simulink model "IOControls"  (R2019b)
settings: configuration reference "ConfigSet_IOControls_Reference" (kept outside this file)
model workspace (MAT data in the model file):
  SampleTime = 0.05
libraries: IOStateMachinesLib x274, SignalGeneratorsLib x1, simulink x1
(part 6 of 10)

== system IOControls/ForEachVehicle/IOControls/Non-CabControl/CircuitBreakersofEDB/ILCB2 ==
  note: States:
      | Tripped
      | Set
  MCBControl : Inport  OutDataTypeStr=Bus: BD_IOControls_In_MCBControl
  Initialise : Inport  Port=2
  Bus Selector : BusSelector  OutputSignals=Value,Mode,InitVal,InternalRequest,Inhibit,TripRequest
  ILCB2-MCB : IOStateMachinesLib/MCB  InitSource=internal  InitState=InitState  OffStateValue=OffStateValue  OnStateValue=OnStateValue
      settings: SourceProductName=IO State Machines
  InputState : Outport  VectorParamsAs1DForOutWhenUnconnected=off
  MCBTripState : Outport  Port=2  VectorParamsAs1DForOutWhenUnconnected=off
  wires:
  ILCB2-MCB/2 -> MCBTripState/1
  Bus Selector/6 -> ILCB2-MCB/7  "<TripRequest>"
  MCBControl/1 -> Bus Selector/1
  Bus Selector/1 -> ILCB2-MCB/1  "<Value>"
  Bus Selector/2 -> ILCB2-MCB/2  "<Mode>"
  Bus Selector/3 -> ILCB2-MCB/3  "<InitVal>"
  Bus Selector/4 -> ILCB2-MCB/5  "<InternalRequest>"
  Bus Selector/5 -> ILCB2-MCB/6  "<Inhibit>"
  ILCB2-MCB/1 -> InputState/1
  Initialise/1 -> ILCB2-MCB/4

== system IOControls/ForEachVehicle/IOControls/Non-CabControl/CircuitBreakersofEDB/LDICB ==
  note: States:
      | Tripped
      | Set
  MCBControl : Inport  OutDataTypeStr=Bus: BD_IOControls_In_MCBControl
  Initialise : Inport  Port=2
  Bus Selector : BusSelector  OutputSignals=Value,Mode,InitVal,InternalRequest,Inhibit,TripRequest
  LDICB-MCB : IOStateMachinesLib/MCB  InitSource=internal  InitState=InitState  OffStateValue=OffStateValue  OnStateValue=OnStateValue
      settings: SourceProductName=IO State Machines
  InputState : Outport  VectorParamsAs1DForOutWhenUnconnected=off
  MCBTripState : Outport  Port=2  VectorParamsAs1DForOutWhenUnconnected=off
  wires:
  LDICB-MCB/2 -> MCBTripState/1
  Bus Selector/6 -> LDICB-MCB/7  "<TripRequest>"
  MCBControl/1 -> Bus Selector/1
  Bus Selector/1 -> LDICB-MCB/1  "<Value>"
  Bus Selector/2 -> LDICB-MCB/2  "<Mode>"
  Bus Selector/3 -> LDICB-MCB/3  "<InitVal>"
  Bus Selector/4 -> LDICB-MCB/5  "<InternalRequest>"
  Bus Selector/5 -> LDICB-MCB/6  "<Inhibit>"
  LDICB-MCB/1 -> InputState/1
  Initialise/1 -> LDICB-MCB/4

== system IOControls/ForEachVehicle/IOControls/Non-CabControl/CircuitBreakersofEDB/LDLCB ==
  note: States:
      | Tripped
      | Set
  MCBControl : Inport  OutDataTypeStr=Bus: BD_IOControls_In_MCBControl
  Initialise : Inport  Port=2
  Bus Selector : BusSelector  OutputSignals=Value,Mode,InitVal,InternalRequest,Inhibit,TripRequest
  LDLCB-MCB : IOStateMachinesLib/MCB  InitSource=internal  InitState=InitState  OffStateValue=OffStateValue  OnStateValue=OnStateValue
      settings: SourceProductName=IO State Machines
  InputState : Outport  VectorParamsAs1DForOutWhenUnconnected=off
  MCBTripState : Outport  Port=2  VectorParamsAs1DForOutWhenUnconnected=off
  wires:
  LDLCB-MCB/2 -> MCBTripState/1
  Bus Selector/6 -> LDLCB-MCB/7  "<TripRequest>"
  MCBControl/1 -> Bus Selector/1
  Bus Selector/1 -> LDLCB-MCB/1  "<Value>"
  Bus Selector/2 -> LDLCB-MCB/2  "<Mode>"
  Bus Selector/3 -> LDLCB-MCB/3  "<InitVal>"
  Bus Selector/4 -> LDLCB-MCB/5  "<InternalRequest>"
  Bus Selector/5 -> LDLCB-MCB/6  "<Inhibit>"
  LDLCB-MCB/1 -> InputState/1
  Initialise/1 -> LDLCB-MCB/4

== system IOControls/ForEachVehicle/IOControls/Non-CabControl/CircuitBreakersofEDB/LDRCB ==
  note: States:
      | Tripped
      | Set
  MCBControl : Inport  OutDataTypeStr=Bus: BD_IOControls_In_MCBControl
  Initialise : Inport  Port=2
  Bus Selector : BusSelector  OutputSignals=Value,Mode,InitVal,InternalRequest,Inhibit,TripRequest
  LDRCB-MCB : IOStateMachinesLib/MCB  InitSource=internal  InitState=InitState  OffStateValue=OffStateValue  OnStateValue=OnStateValue
      settings: SourceProductName=IO State Machines
  InputState : Outport  VectorParamsAs1DForOutWhenUnconnected=off
  MCBTripState : Outport  Port=2  VectorParamsAs1DForOutWhenUnconnected=off
  wires:
  LDRCB-MCB/2 -> MCBTripState/1
  Bus Selector/6 -> LDRCB-MCB/7  "<TripRequest>"
  MCBControl/1 -> Bus Selector/1
  Bus Selector/1 -> LDRCB-MCB/1  "<Value>"
  Bus Selector/2 -> LDRCB-MCB/2  "<Mode>"
  Bus Selector/3 -> LDRCB-MCB/3  "<InitVal>"
  Bus Selector/4 -> LDRCB-MCB/5  "<InternalRequest>"
  Bus Selector/5 -> LDRCB-MCB/6  "<Inhibit>"
  LDRCB-MCB/1 -> InputState/1
  Initialise/1 -> LDRCB-MCB/4

== system IOControls/ForEachVehicle/IOControls/Non-CabControl/CircuitBreakersofEDB/MLCB ==
  note: States:
      | Tripped
      | Set
  MCBControl : Inport  OutDataTypeStr=Bus: BD_IOControls_In_MCBControl
  Initialise : Inport  Port=2
  Bus Selector : BusSelector  OutputSignals=Value,Mode,InitVal,InternalRequest,Inhibit,TripRequest
  MLCB-MCB : IOStateMachinesLib/MCB  InitSource=internal  InitState=InitState  OffStateValue=OffStateValue  OnStateValue=OnStateValue
      settings: SourceProductName=IO State Machines
  InputState : Outport  VectorParamsAs1DForOutWhenUnconnected=off
  MCBTripState : Outport  Port=2  VectorParamsAs1DForOutWhenUnconnected=off
  wires:
  MLCB-MCB/2 -> MCBTripState/1
  Bus Selector/6 -> MLCB-MCB/7  "<TripRequest>"
  MCBControl/1 -> Bus Selector/1
  Bus Selector/1 -> MLCB-MCB/1  "<Value>"
  Bus Selector/2 -> MLCB-MCB/2  "<Mode>"
  Bus Selector/3 -> MLCB-MCB/3  "<InitVal>"
  Bus Selector/4 -> MLCB-MCB/5  "<InternalRequest>"
  Bus Selector/5 -> MLCB-MCB/6  "<Inhibit>"
  MLCB-MCB/1 -> InputState/1
  Initialise/1 -> MLCB-MCB/4

== system IOControls/ForEachVehicle/IOControls/Non-CabControl/CircuitBreakersofEDB/MMCB ==
  note: States:
      | Tripped
      | Set
  MCBControl : Inport  OutDataTypeStr=Bus: BD_IOControls_In_MCBControl
  Initialise : Inport  Port=2
  Bus Selector : BusSelector  OutputSignals=Value,Mode,InitVal,InternalRequest,Inhibit,TripRequest
  MMCB-MCB : IOStateMachinesLib/MCB  InitSource=internal  InitState=InitState  OffStateValue=OffStateValue  OnStateValue=OnStateValue
      settings: SourceProductName=IO State Machines
  InputState : Outport  VectorParamsAs1DForOutWhenUnconnected=off
  MCBTripState : Outport  Port=2  VectorParamsAs1DForOutWhenUnconnected=off
  wires:
  MMCB-MCB/2 -> MCBTripState/1
  Bus Selector/6 -> MMCB-MCB/7  "<TripRequest>"
  MCBControl/1 -> Bus Selector/1
  Bus Selector/1 -> MMCB-MCB/1  "<Value>"
  Bus Selector/2 -> MMCB-MCB/2  "<Mode>"
  Bus Selector/3 -> MMCB-MCB/3  "<InitVal>"
  Bus Selector/4 -> MMCB-MCB/5  "<InternalRequest>"
  Bus Selector/5 -> MMCB-MCB/6  "<Inhibit>"
  MMCB-MCB/1 -> InputState/1
  Initialise/1 -> MMCB-MCB/4

== system IOControls/ForEachVehicle/IOControls/Non-CabControl/CircuitBreakersofEDB/MSOCB1 ==
  note: States:
      | Tripped
      | Set
  MCBControl : Inport  OutDataTypeStr=Bus: BD_IOControls_In_MCBControl
  Initialise : Inport  Port=2
  Bus Selector : BusSelector  OutputSignals=Value,Mode,InitVal,InternalRequest,Inhibit,TripRequest
  MSOCB1-MCB : IOStateMachinesLib/MCB  InitSource=internal  InitState=InitState  OffStateValue=OffStateValue  OnStateValue=OnStateValue
      settings: SourceProductName=IO State Machines
  InputState : Outport  VectorParamsAs1DForOutWhenUnconnected=off
  MCBTripState : Outport  Port=2  VectorParamsAs1DForOutWhenUnconnected=off
  wires:
  MSOCB1-MCB/2 -> MCBTripState/1
  Bus Selector/6 -> MSOCB1-MCB/7  "<TripRequest>"
  MCBControl/1 -> Bus Selector/1
  Bus Selector/1 -> MSOCB1-MCB/1  "<Value>"
  Bus Selector/2 -> MSOCB1-MCB/2  "<Mode>"
  Bus Selector/3 -> MSOCB1-MCB/3  "<InitVal>"
  Bus Selector/4 -> MSOCB1-MCB/5  "<InternalRequest>"
  Bus Selector/5 -> MSOCB1-MCB/6  "<Inhibit>"
  MSOCB1-MCB/1 -> InputState/1
  Initialise/1 -> MSOCB1-MCB/4

== system IOControls/ForEachVehicle/IOControls/Non-CabControl/CircuitBreakersofEDB/MSOCB2 ==
  note: States:
      | Tripped
      | Set
  MCBControl : Inport  OutDataTypeStr=Bus: BD_IOControls_In_MCBControl
  Initialise : Inport  Port=2
  Bus Selector : BusSelector  OutputSignals=Value,Mode,InitVal,InternalRequest,Inhibit,TripRequest
  MSOCB2-MCB : IOStateMachinesLib/MCB  InitSource=internal  InitState=InitState  OffStateValue=OffStateValue  OnStateValue=OnStateValue
      settings: SourceProductName=IO State Machines
  InputState : Outport  VectorParamsAs1DForOutWhenUnconnected=off
  MCBTripState : Outport  Port=2  VectorParamsAs1DForOutWhenUnconnected=off
  wires:
  MSOCB2-MCB/2 -> MCBTripState/1
  Bus Selector/6 -> MSOCB2-MCB/7  "<TripRequest>"
  MCBControl/1 -> Bus Selector/1
  Bus Selector/1 -> MSOCB2-MCB/1  "<Value>"
  Bus Selector/2 -> MSOCB2-MCB/2  "<Mode>"
  Bus Selector/3 -> MSOCB2-MCB/3  "<InitVal>"
  Bus Selector/4 -> MSOCB2-MCB/5  "<InternalRequest>"
  Bus Selector/5 -> MSOCB2-MCB/6  "<Inhibit>"
  MSOCB2-MCB/1 -> InputState/1
  Initialise/1 -> MSOCB2-MCB/4

== system IOControls/ForEachVehicle/IOControls/Non-CabControl/CircuitBreakersofEDB/MSOCB3 ==
  note: States:
      | Tripped
      | Set
  MCBControl : Inport  OutDataTypeStr=Bus: BD_IOControls_In_MCBControl
  Initialise : Inport  Port=2
  Bus Selector : BusSelector  OutputSignals=Value,Mode,InitVal,InternalRequest,Inhibit,TripRequest
  MSOCB3-MCB : IOStateMachinesLib/MCB  InitSource=internal  InitState=InitState  OffStateValue=OffStateValue  OnStateValue=OnStateValue
      settings: SourceProductName=IO State Machines
  InputState : Outport  VectorParamsAs1DForOutWhenUnconnected=off
  MCBTripState : Outport  Port=2  VectorParamsAs1DForOutWhenUnconnected=off
  wires:
  MSOCB3-MCB/2 -> MCBTripState/1
  Bus Selector/6 -> MSOCB3-MCB/7  "<TripRequest>"
  MCBControl/1 -> Bus Selector/1
  Bus Selector/1 -> MSOCB3-MCB/1  "<Value>"
  Bus Selector/2 -> MSOCB3-MCB/2  "<Mode>"
  Bus Selector/3 -> MSOCB3-MCB/3  "<InitVal>"
  Bus Selector/4 -> MSOCB3-MCB/5  "<InternalRequest>"
  Bus Selector/5 -> MSOCB3-MCB/6  "<Inhibit>"
  MSOCB3-MCB/1 -> InputState/1
  Initialise/1 -> MSOCB3-MCB/4

== system IOControls/ForEachVehicle/IOControls/Non-CabControl/CircuitBreakersofEDB/MSOCB4 ==
  note: States:
      | Tripped
      | Set
  MCBControl : Inport  OutDataTypeStr=Bus: BD_IOControls_In_MCBControl
  Initialise : Inport  Port=2
  Bus Selector : BusSelector  OutputSignals=Value,Mode,InitVal,InternalRequest,Inhibit,TripRequest
  MSOCB4-MCB : IOStateMachinesLib/MCB  InitSource=internal  InitState=InitState  OffStateValue=OffStateValue  OnStateValue=OnStateValue
      settings: SourceProductName=IO State Machines
  InputState : Outport  VectorParamsAs1DForOutWhenUnconnected=off
  MCBTripState : Outport  Port=2  VectorParamsAs1DForOutWhenUnconnected=off
  wires:
  MSOCB4-MCB/2 -> MCBTripState/1
  Bus Selector/6 -> MSOCB4-MCB/7  "<TripRequest>"
  MCBControl/1 -> Bus Selector/1
  Bus Selector/1 -> MSOCB4-MCB/1  "<Value>"
  Bus Selector/2 -> MSOCB4-MCB/2  "<Mode>"
  Bus Selector/3 -> MSOCB4-MCB/3  "<InitVal>"
  Bus Selector/4 -> MSOCB4-MCB/5  "<InternalRequest>"
  Bus Selector/5 -> MSOCB4-MCB/6  "<Inhibit>"
  MSOCB4-MCB/1 -> InputState/1
  Initialise/1 -> MSOCB4-MCB/4

== system IOControls/ForEachVehicle/IOControls/Non-CabControl/CircuitBreakersofEDB/MSOCB5 ==
  note: States:
      | Tripped
      | Set
  MCBControl : Inport  OutDataTypeStr=Bus: BD_IOControls_In_MCBControl
  Initialise : Inport  Port=2
  Bus Selector : BusSelector  OutputSignals=Value,Mode,InitVal,InternalRequest,Inhibit,TripRequest
  MSOCB5-MCB : IOStateMachinesLib/MCB  InitSource=internal  InitState=InitState  OffStateValue=OffStateValue  OnStateValue=OnStateValue
      settings: SourceProductName=IO State Machines
  InputState : Outport  VectorParamsAs1DForOutWhenUnconnected=off
  MCBTripState : Outport  Port=2  VectorParamsAs1DForOutWhenUnconnected=off
  wires:
  MSOCB5-MCB/2 -> MCBTripState/1
  Bus Selector/6 -> MSOCB5-MCB/7  "<TripRequest>"
  MCBControl/1 -> Bus Selector/1
  Bus Selector/1 -> MSOCB5-MCB/1  "<Value>"
  Bus Selector/2 -> MSOCB5-MCB/2  "<Mode>"
  Bus Selector/3 -> MSOCB5-MCB/3  "<InitVal>"
  Bus Selector/4 -> MSOCB5-MCB/5  "<InternalRequest>"
  Bus Selector/5 -> MSOCB5-MCB/6  "<Inhibit>"
  MSOCB5-MCB/1 -> InputState/1
  Initialise/1 -> MSOCB5-MCB/4

== system IOControls/ForEachVehicle/IOControls/Non-CabControl/CircuitBreakersofEDB/MTBM1CB ==
  note: States:
      | Tripped
      | Set
  MCBControl : Inport  OutDataTypeStr=Bus: BD_IOControls_In_MCBControl
  Initialise : Inport  Port=2
  Bus Selector : BusSelector  OutputSignals=Value,Mode,InitVal,InternalRequest,Inhibit,TripRequest
  MTBM1CB-MCB : IOStateMachinesLib/MCB  InitSource=internal  InitState=InitState  OffStateValue=OffStateValue  OnStateValue=OnStateValue
      settings: SourceProductName=IO State Machines
  InputState : Outport  VectorParamsAs1DForOutWhenUnconnected=off
  MCBTripState : Outport  Port=2  VectorParamsAs1DForOutWhenUnconnected=off
  wires:
  MTBM1CB-MCB/2 -> MCBTripState/1
  Bus Selector/6 -> MTBM1CB-MCB/7  "<TripRequest>"
  MCBControl/1 -> Bus Selector/1
  Bus Selector/1 -> MTBM1CB-MCB/1  "<Value>"
  Bus Selector/2 -> MTBM1CB-MCB/2  "<Mode>"
  Bus Selector/3 -> MTBM1CB-MCB/3  "<InitVal>"
  Bus Selector/4 -> MTBM1CB-MCB/5  "<InternalRequest>"
  Bus Selector/5 -> MTBM1CB-MCB/6  "<Inhibit>"
  MTBM1CB-MCB/1 -> InputState/1
  Initialise/1 -> MTBM1CB-MCB/4

== system IOControls/ForEachVehicle/IOControls/Non-CabControl/CircuitBreakersofEDB/MTBM2CB ==
  note: States:
      | Tripped
      | Set
  MCBControl : Inport  OutDataTypeStr=Bus: BD_IOControls_In_MCBControl
  Initialise : Inport  Port=2
  Bus Selector : BusSelector  OutputSignals=Value,Mode,InitVal,InternalRequest,Inhibit,TripRequest
  MTBM2CB-MCB : IOStateMachinesLib/MCB  InitSource=internal  InitState=InitState  OffStateValue=OffStateValue  OnStateValue=OnStateValue
      settings: SourceProductName=IO State Machines
  InputState : Outport  VectorParamsAs1DForOutWhenUnconnected=off
  MCBTripState : Outport  Port=2  VectorParamsAs1DForOutWhenUnconnected=off
  wires:
  MTBM2CB-MCB/2 -> MCBTripState/1
  Bus Selector/6 -> MTBM2CB-MCB/7  "<TripRequest>"
  MCBControl/1 -> Bus Selector/1
  Bus Selector/1 -> MTBM2CB-MCB/1  "<Value>"
  Bus Selector/2 -> MTBM2CB-MCB/2  "<Mode>"
  Bus Selector/3 -> MTBM2CB-MCB/3  "<InitVal>"
  Bus Selector/4 -> MTBM2CB-MCB/5  "<InternalRequest>"
  Bus Selector/5 -> MTBM2CB-MCB/6  "<Inhibit>"
  MTBM2CB-MCB/1 -> InputState/1
  Initialise/1 -> MTBM2CB-MCB/4

== system IOControls/ForEachVehicle/IOControls/Non-CabControl/CircuitBreakersofEDB/MTBMCCB ==
  note: States:
      | Tripped
      | Set
  MCBControl : Inport  OutDataTypeStr=Bus: BD_IOControls_In_MCBControl
  Initialise : Inport  Port=2
  Bus Selector : BusSelector  OutputSignals=Value,Mode,InitVal,InternalRequest,Inhibit,TripRequest
  MTBMCCB-MCB : IOStateMachinesLib/MCB  InitSource=internal  InitState=InitState  OffStateValue=OffStateValue  OnStateValue=OnStateValue
      settings: SourceProductName=IO State Machines
  InputState : Outport  VectorParamsAs1DForOutWhenUnconnected=off
  MCBTripState : Outport  Port=2  VectorParamsAs1DForOutWhenUnconnected=off
  wires:
  MTBMCCB-MCB/2 -> MCBTripState/1
  Bus Selector/6 -> MTBMCCB-MCB/7  "<TripRequest>"
  MCBControl/1 -> Bus Selector/1
  Bus Selector/1 -> MTBMCCB-MCB/1  "<Value>"
  Bus Selector/2 -> MTBMCCB-MCB/2  "<Mode>"
  Bus Selector/3 -> MTBMCCB-MCB/3  "<InitVal>"
  Bus Selector/4 -> MTBMCCB-MCB/5  "<InternalRequest>"
  Bus Selector/5 -> MTBMCCB-MCB/6  "<Inhibit>"
  MTBMCCB-MCB/1 -> InputState/1
  Initialise/1 -> MTBMCCB-MCB/4

== system IOControls/ForEachVehicle/IOControls/Non-CabControl/CircuitBreakersofEDB/MTOPCB ==
  note: States:
      | Tripped
      | Set
  MCBControl : Inport  OutDataTypeStr=Bus: BD_IOControls_In_MCBControl
  Initialise : Inport  Port=2
  Bus Selector : BusSelector  OutputSignals=Value,Mode,InitVal,InternalRequest,Inhibit,TripRequest
  MTOPCB-MCB : IOStateMachinesLib/MCB  InitSource=internal  InitState=InitState  OffStateValue=OffStateValue  OnStateValue=OnStateValue
      settings: SourceProductName=IO State Machines
  InputState : Outport  VectorParamsAs1DForOutWhenUnconnected=off
  MCBTripState : Outport  Port=2  VectorParamsAs1DForOutWhenUnconnected=off
  wires:
  MTOPCB-MCB/2 -> MCBTripState/1
  Bus Selector/6 -> MTOPCB-MCB/7  "<TripRequest>"
  MCBControl/1 -> Bus Selector/1
  Bus Selector/1 -> MTOPCB-MCB/1  "<Value>"
  Bus Selector/2 -> MTOPCB-MCB/2  "<Mode>"
  Bus Selector/3 -> MTOPCB-MCB/3  "<InitVal>"
  Bus Selector/4 -> MTOPCB-MCB/5  "<InternalRequest>"
  Bus Selector/5 -> MTOPCB-MCB/6  "<Inhibit>"
  MTOPCB-MCB/1 -> InputState/1
  Initialise/1 -> MTOPCB-MCB/4

== system IOControls/ForEachVehicle/IOControls/Non-CabControl/CircuitBreakersofEDB/NBCB ==
  note: States:
      | Tripped
      | Set
  MCBControl : Inport  OutDataTypeStr=Bus: BD_IOControls_In_MCBControl
  Initialise : Inport  Port=2
  Bus Selector : BusSelector  OutputSignals=Value,Mode,InitVal,InternalRequest,Inhibit,TripRequest
  NBCB-MCB : IOStateMachinesLib/MCB  InitSource=internal  InitState=InitState  OffStateValue=OffStateValue  OnStateValue=OnStateValue
      settings: SourceProductName=IO State Machines
  InputState : Outport  VectorParamsAs1DForOutWhenUnconnected=off
  MCBTripState : Outport  Port=2  VectorParamsAs1DForOutWhenUnconnected=off
  wires:
  NBCB-MCB/2 -> MCBTripState/1
  Bus Selector/6 -> NBCB-MCB/7  "<TripRequest>"
  MCBControl/1 -> Bus Selector/1
  Bus Selector/1 -> NBCB-MCB/1  "<Value>"
  Bus Selector/2 -> NBCB-MCB/2  "<Mode>"
  Bus Selector/3 -> NBCB-MCB/3  "<InitVal>"
  Bus Selector/4 -> NBCB-MCB/5  "<InternalRequest>"
  Bus Selector/5 -> NBCB-MCB/6  "<Inhibit>"
  NBCB-MCB/1 -> InputState/1
  Initialise/1 -> NBCB-MCB/4

== system IOControls/ForEachVehicle/IOControls/Non-CabControl/CircuitBreakersofEDB/NVICB ==
  note: States:
      | Tripped
      | Set
  MCBControl : Inport  OutDataTypeStr=Bus: BD_IOControls_In_MCBControl
  Initialise : Inport  Port=2
  Bus Selector : BusSelector  OutputSignals=Value,Mode,InitVal,InternalRequest,Inhibit,TripRequest
  NVICB-MCB : IOStateMachinesLib/MCB  InitSource=internal  InitState=InitState  OffStateValue=OffStateValue  OnStateValue=OnStateValue
      settings: SourceProductName=IO State Machines
  InputState : Outport  VectorParamsAs1DForOutWhenUnconnected=off
  MCBTripState : Outport  Port=2  VectorParamsAs1DForOutWhenUnconnected=off
  wires:
  NVICB-MCB/2 -> MCBTripState/1
  Bus Selector/6 -> NVICB-MCB/7  "<TripRequest>"
  MCBControl/1 -> Bus Selector/1
  Bus Selector/1 -> NVICB-MCB/1  "<Value>"
  Bus Selector/2 -> NVICB-MCB/2  "<Mode>"
  Bus Selector/3 -> NVICB-MCB/3  "<InitVal>"
  Bus Selector/4 -> NVICB-MCB/5  "<InternalRequest>"
  Bus Selector/5 -> NVICB-MCB/6  "<Inhibit>"
  NVICB-MCB/1 -> InputState/1
  Initialise/1 -> NVICB-MCB/4

== system IOControls/ForEachVehicle/IOControls/Non-CabControl/CircuitBreakersofEDB/OCCB1 ==
  note: States:
      | Tripped
      | Set
  MCBControl : Inport  OutDataTypeStr=Bus: BD_IOControls_In_MCBControl
  Initialise : Inport  Port=2
  Bus Selector : BusSelector  OutputSignals=Value,Mode,InitVal,InternalRequest,Inhibit,TripRequest
  OCCB1-MCB : IOStateMachinesLib/MCB  InitSource=internal  InitState=InitState  OffStateValue=OffStateValue  OnStateValue=OnStateValue
      settings: SourceProductName=IO State Machines
  InputState : Outport  VectorParamsAs1DForOutWhenUnconnected=off
  MCBTripState : Outport  Port=2  VectorParamsAs1DForOutWhenUnconnected=off
  wires:
  OCCB1-MCB/2 -> MCBTripState/1
  Bus Selector/6 -> OCCB1-MCB/7  "<TripRequest>"
  MCBControl/1 -> Bus Selector/1
  Bus Selector/1 -> OCCB1-MCB/1  "<Value>"
  Bus Selector/2 -> OCCB1-MCB/2  "<Mode>"
  Bus Selector/3 -> OCCB1-MCB/3  "<InitVal>"
  Bus Selector/4 -> OCCB1-MCB/5  "<InternalRequest>"
  Bus Selector/5 -> OCCB1-MCB/6  "<Inhibit>"
  OCCB1-MCB/1 -> InputState/1
  Initialise/1 -> OCCB1-MCB/4

== system IOControls/ForEachVehicle/IOControls/Non-CabControl/CircuitBreakersofEDB/OCCB2 ==
  note: States:
      | Tripped
      | Set
  MCBControl : Inport  OutDataTypeStr=Bus: BD_IOControls_In_MCBControl
  Initialise : Inport  Port=2
  Bus Selector : BusSelector  OutputSignals=Value,Mode,InitVal,InternalRequest,Inhibit,TripRequest
  OCCB2-MCB : IOStateMachinesLib/MCB  InitSource=internal  InitState=InitState  OffStateValue=OffStateValue  OnStateValue=OnStateValue
      settings: SourceProductName=IO State Machines
  InputState : Outport  VectorParamsAs1DForOutWhenUnconnected=off
  MCBTripState : Outport  Port=2  VectorParamsAs1DForOutWhenUnconnected=off
  wires:
  OCCB2-MCB/2 -> MCBTripState/1
  Bus Selector/6 -> OCCB2-MCB/7  "<TripRequest>"
  MCBControl/1 -> Bus Selector/1
  Bus Selector/1 -> OCCB2-MCB/1  "<Value>"
  Bus Selector/2 -> OCCB2-MCB/2  "<Mode>"
  Bus Selector/3 -> OCCB2-MCB/3  "<InitVal>"
  Bus Selector/4 -> OCCB2-MCB/5  "<InternalRequest>"
  Bus Selector/5 -> OCCB2-MCB/6  "<Inhibit>"
  OCCB2-MCB/1 -> InputState/1
  Initialise/1 -> OCCB2-MCB/4

== system IOControls/ForEachVehicle/IOControls/Non-CabControl/CircuitBreakersofEDB/ODDCB ==
  note: States:
      | Tripped
      | Set
  MCBControl : Inport  OutDataTypeStr=Bus: BD_IOControls_In_MCBControl
  Initialise : Inport  Port=2
  Bus Selector : BusSelector  OutputSignals=Value,Mode,InitVal,InternalRequest,Inhibit,TripRequest
  ODDCB-MCB : IOStateMachinesLib/MCB  InitSource=internal  InitState=InitState  OffStateValue=OffStateValue  OnStateValue=OnStateValue
      settings: SourceProductName=IO State Machines
  InputState : Outport  VectorParamsAs1DForOutWhenUnconnected=off
  MCBTripState : Outport  Port=2  VectorParamsAs1DForOutWhenUnconnected=off
  wires:
  ODDCB-MCB/2 -> MCBTripState/1
  Bus Selector/6 -> ODDCB-MCB/7  "<TripRequest>"
  MCBControl/1 -> Bus Selector/1
  Bus Selector/1 -> ODDCB-MCB/1  "<Value>"
  Bus Selector/2 -> ODDCB-MCB/2  "<Mode>"
  Bus Selector/3 -> ODDCB-MCB/3  "<InitVal>"
  Bus Selector/4 -> ODDCB-MCB/5  "<InternalRequest>"
  Bus Selector/5 -> ODDCB-MCB/6  "<Inhibit>"
  ODDCB-MCB/1 -> InputState/1
  Initialise/1 -> ODDCB-MCB/4

== system IOControls/ForEachVehicle/IOControls/Non-CabControl/CircuitBreakersofEDB/ORDCOS ==
  note: States:
      | Normal
      | Cutout
  InputControl : Inport  OutDataTypeStr=Bus: BD_IOControls_In_InputControl
  Initialise : Inport  Port=2
  Bus Selector : BusSelector  OutputSignals=Value,Mode,InitVal,InternalRequest,Inhibit
  ORDCOS-Toggle : IOStateMachinesLib/Toggle  InitSource=internal  InitState=InitState  OffStateValue=OffStateValue  OnStateValue=OnStateValue
      settings: SourceProductName=IO State Machines
  InputState : Outport  VectorParamsAs1DForOutWhenUnconnected=off
  wires:
  Initialise/1 -> ORDCOS-Toggle/4
  ORDCOS-Toggle/1 -> InputState/1
  Bus Selector/5 -> ORDCOS-Toggle/6  "<Inhibit>"
  Bus Selector/4 -> ORDCOS-Toggle/5  "<InternalRequest>"
  Bus Selector/3 -> ORDCOS-Toggle/3  "<InitVal>"
  Bus Selector/2 -> ORDCOS-Toggle/2  "<Mode>"
  Bus Selector/1 -> ORDCOS-Toggle/1  "<Value>"
  InputControl/1 -> Bus Selector/1

== system IOControls/ForEachVehicle/IOControls/Non-CabControl/CircuitBreakersofEDB/PADCB ==
  note: States:
      | Tripped
      | Set
  MCBControl : Inport  OutDataTypeStr=Bus: BD_IOControls_In_MCBControl
  Initialise : Inport  Port=2
  Bus Selector : BusSelector  OutputSignals=Value,Mode,InitVal,InternalRequest,Inhibit,TripRequest
  PADCB-MCB : IOStateMachinesLib/MCB  InitSource=internal  InitState=InitState  OffStateValue=OffStateValue  OnStateValue=OnStateValue
      settings: SourceProductName=IO State Machines
  InputState : Outport  VectorParamsAs1DForOutWhenUnconnected=off
  MCBTripState : Outport  Port=2  VectorParamsAs1DForOutWhenUnconnected=off
  wires:
  PADCB-MCB/2 -> MCBTripState/1
  Bus Selector/6 -> PADCB-MCB/7  "<TripRequest>"
  MCBControl/1 -> Bus Selector/1
  Bus Selector/1 -> PADCB-MCB/1  "<Value>"
  Bus Selector/2 -> PADCB-MCB/2  "<Mode>"
  Bus Selector/3 -> PADCB-MCB/3  "<InitVal>"
  Bus Selector/4 -> PADCB-MCB/5  "<InternalRequest>"
  Bus Selector/5 -> PADCB-MCB/6  "<Inhibit>"
  PADCB-MCB/1 -> InputState/1
  Initialise/1 -> PADCB-MCB/4

== system IOControls/ForEachVehicle/IOControls/Non-CabControl/CircuitBreakersofEDB/PANCB ==
  note: States:
      | Tripped
      | Set
  MCBControl : Inport  OutDataTypeStr=Bus: BD_IOControls_In_MCBControl
  Initialise : Inport  Port=2
  Bus Selector : BusSelector  OutputSignals=Value,Mode,InitVal,InternalRequest,Inhibit,TripRequest
  PANCB-MCB : IOStateMachinesLib/MCB  InitSource=internal  InitState=InitState  OffStateValue=OffStateValue  OnStateValue=OnStateValue
      settings: SourceProductName=IO State Machines
  InputState : Outport  VectorParamsAs1DForOutWhenUnconnected=off
  MCBTripState : Outport  Port=2  VectorParamsAs1DForOutWhenUnconnected=off
  wires:
  PANCB-MCB/2 -> MCBTripState/1
  Bus Selector/6 -> PANCB-MCB/7  "<TripRequest>"
  MCBControl/1 -> Bus Selector/1
  Bus Selector/1 -> PANCB-MCB/1  "<Value>"
  Bus Selector/2 -> PANCB-MCB/2  "<Mode>"
  Bus Selector/3 -> PANCB-MCB/3  "<InitVal>"
  Bus Selector/4 -> PANCB-MCB/5  "<InternalRequest>"
  Bus Selector/5 -> PANCB-MCB/6  "<Inhibit>"
  PANCB-MCB/1 -> InputState/1
  Initialise/1 -> PANCB-MCB/4

== system IOControls/ForEachVehicle/IOControls/Non-CabControl/CircuitBreakersofEDB/PBCB ==
  note: States:
      | Tripped
      | Set
  MCBControl : Inport  OutDataTypeStr=Bus: BD_IOControls_In_MCBControl
  Initialise : Inport  Port=2
  Bus Selector : BusSelector  OutputSignals=Value,Mode,InitVal,InternalRequest,Inhibit,TripRequest
  PBCB-MCB : IOStateMachinesLib/MCB  InitSource=internal  InitState=InitState  OffStateValue=OffStateValue  OnStateValue=OnStateValue
      settings: SourceProductName=IO State Machines
  InputState : Outport  VectorParamsAs1DForOutWhenUnconnected=off
  MCBTripState : Outport  Port=2  VectorParamsAs1DForOutWhenUnconnected=off
  wires:
  PBCB-MCB/2 -> MCBTripState/1
  Bus Selector/6 -> PBCB-MCB/7  "<TripRequest>"
  MCBControl/1 -> Bus Selector/1
  Bus Selector/1 -> PBCB-MCB/1  "<Value>"
  Bus Selector/2 -> PBCB-MCB/2  "<Mode>"
  Bus Selector/3 -> PBCB-MCB/3  "<InitVal>"
  Bus Selector/4 -> PBCB-MCB/5  "<InternalRequest>"
  Bus Selector/5 -> PBCB-MCB/6  "<Inhibit>"
  PBCB-MCB/1 -> InputState/1
  Initialise/1 -> PBCB-MCB/4

== system IOControls/ForEachVehicle/IOControls/Non-CabControl/CircuitBreakersofEDB/PISCB1 ==
  note: States:
      | Tripped
      | Set
  MCBControl : Inport  OutDataTypeStr=Bus: BD_IOControls_In_MCBControl
  Initialise : Inport  Port=2
  Bus Selector : BusSelector  OutputSignals=Value,Mode,InitVal,InternalRequest,Inhibit,TripRequest
  PISCB1-MCB : IOStateMachinesLib/MCB  InitSource=internal  InitState=InitState  OffStateValue=OffStateValue  OnStateValue=OnStateValue
      settings: SourceProductName=IO State Machines
  InputState : Outport  VectorParamsAs1DForOutWhenUnconnected=off
  MCBTripState : Outport  Port=2  VectorParamsAs1DForOutWhenUnconnected=off
  wires:
  PISCB1-MCB/2 -> MCBTripState/1
  Bus Selector/6 -> PISCB1-MCB/7  "<TripRequest>"
  MCBControl/1 -> Bus Selector/1
  Bus Selector/1 -> PISCB1-MCB/1  "<Value>"
  Bus Selector/2 -> PISCB1-MCB/2  "<Mode>"
  Bus Selector/3 -> PISCB1-MCB/3  "<InitVal>"
  Bus Selector/4 -> PISCB1-MCB/5  "<InternalRequest>"
  Bus Selector/5 -> PISCB1-MCB/6  "<Inhibit>"
  PISCB1-MCB/1 -> InputState/1
  Initialise/1 -> PISCB1-MCB/4

== system IOControls/ForEachVehicle/IOControls/Non-CabControl/CircuitBreakersofEDB/PISCB2 ==
  note: States:
      | Tripped
      | Set
  MCBControl : Inport  OutDataTypeStr=Bus: BD_IOControls_In_MCBControl
  Initialise : Inport  Port=2
  Bus Selector : BusSelector  OutputSignals=Value,Mode,InitVal,InternalRequest,Inhibit,TripRequest
  PISCB2-MCB : IOStateMachinesLib/MCB  InitSource=internal  InitState=InitState  OffStateValue=OffStateValue  OnStateValue=OnStateValue
      settings: SourceProductName=IO State Machines
  InputState : Outport  VectorParamsAs1DForOutWhenUnconnected=off
  MCBTripState : Outport  Port=2  VectorParamsAs1DForOutWhenUnconnected=off
  wires:
  PISCB2-MCB/2 -> MCBTripState/1
  Bus Selector/6 -> PISCB2-MCB/7  "<TripRequest>"
  MCBControl/1 -> Bus Selector/1
  Bus Selector/1 -> PISCB2-MCB/1  "<Value>"
  Bus Selector/2 -> PISCB2-MCB/2  "<Mode>"
  Bus Selector/3 -> PISCB2-MCB/3  "<InitVal>"
  Bus Selector/4 -> PISCB2-MCB/5  "<InternalRequest>"
  Bus Selector/5 -> PISCB2-MCB/6  "<Inhibit>"
  PISCB2-MCB/1 -> InputState/1
  Initialise/1 -> PISCB2-MCB/4

== system IOControls/ForEachVehicle/IOControls/Non-CabControl/CircuitBreakersofEDB/POCB ==
  note: States:
      | Tripped
      | Set
  MCBControl : Inport  OutDataTypeStr=Bus: BD_IOControls_In_MCBControl
  Initialise : Inport  Port=2
  Bus Selector : BusSelector  OutputSignals=Value,Mode,InitVal,InternalRequest,Inhibit,TripRequest
  POCB-MCB : IOStateMachinesLib/MCB  InitSource=internal  InitState=InitState  OffStateValue=OffStateValue  OnStateValue=OnStateValue
      settings: SourceProductName=IO State Machines
  InputState : Outport  VectorParamsAs1DForOutWhenUnconnected=off
  MCBTripState : Outport  Port=2  VectorParamsAs1DForOutWhenUnconnected=off
  wires:
  POCB-MCB/2 -> MCBTripState/1
  Bus Selector/6 -> POCB-MCB/7  "<TripRequest>"
  MCBControl/1 -> Bus Selector/1
  Bus Selector/1 -> POCB-MCB/1  "<Value>"
  Bus Selector/2 -> POCB-MCB/2  "<Mode>"
  Bus Selector/3 -> POCB-MCB/3  "<InitVal>"
  Bus Selector/4 -> POCB-MCB/5  "<InternalRequest>"
  Bus Selector/5 -> POCB-MCB/6  "<Inhibit>"
  POCB-MCB/1 -> InputState/1
  Initialise/1 -> POCB-MCB/4

== system IOControls/ForEachVehicle/IOControls/Non-CabControl/CircuitBreakersofEDB/PPU1CB ==
  note: States:
      | Tripped
      | Set
  MCBControl : Inport  OutDataTypeStr=Bus: BD_IOControls_In_MCBControl
  Initialise : Inport  Port=2
  Bus Selector : BusSelector  OutputSignals=Value,Mode,InitVal,InternalRequest,Inhibit,TripRequest
  PPU1CB-MCB : IOStateMachinesLib/MCB  InitSource=internal  InitState=InitState  OffStateValue=OffStateValue  OnStateValue=OnStateValue
      settings: SourceProductName=IO State Machines
  InputState : Outport  VectorParamsAs1DForOutWhenUnconnected=off
  MCBTripState : Outport  Port=2  VectorParamsAs1DForOutWhenUnconnected=off
  wires:
  PPU1CB-MCB/2 -> MCBTripState/1
  Bus Selector/6 -> PPU1CB-MCB/7  "<TripRequest>"
  MCBControl/1 -> Bus Selector/1
  Bus Selector/1 -> PPU1CB-MCB/1  "<Value>"
  Bus Selector/2 -> PPU1CB-MCB/2  "<Mode>"
  Bus Selector/3 -> PPU1CB-MCB/3  "<InitVal>"
  Bus Selector/4 -> PPU1CB-MCB/5  "<InternalRequest>"
  Bus Selector/5 -> PPU1CB-MCB/6  "<Inhibit>"
  PPU1CB-MCB/1 -> InputState/1
  Initialise/1 -> PPU1CB-MCB/4

== system IOControls/ForEachVehicle/IOControls/Non-CabControl/CircuitBreakersofEDB/PPU2CB ==
  note: States:
      | Tripped
      | Set
  MCBControl : Inport  OutDataTypeStr=Bus: BD_IOControls_In_MCBControl
  Initialise : Inport  Port=2
  Bus Selector : BusSelector  OutputSignals=Value,Mode,InitVal,InternalRequest,Inhibit,TripRequest
  PPU2CB-MCB : IOStateMachinesLib/MCB  InitSource=internal  InitState=InitState  OffStateValue=OffStateValue  OnStateValue=OnStateValue
      settings: SourceProductName=IO State Machines
  InputState : Outport  VectorParamsAs1DForOutWhenUnconnected=off
  MCBTripState : Outport  Port=2  VectorParamsAs1DForOutWhenUnconnected=off
  wires:
  PPU2CB-MCB/2 -> MCBTripState/1
  Bus Selector/6 -> PPU2CB-MCB/7  "<TripRequest>"
  MCBControl/1 -> Bus Selector/1
  Bus Selector/1 -> PPU2CB-MCB/1  "<Value>"
  Bus Selector/2 -> PPU2CB-MCB/2  "<Mode>"
  Bus Selector/3 -> PPU2CB-MCB/3  "<InitVal>"
  Bus Selector/4 -> PPU2CB-MCB/5  "<InternalRequest>"
  Bus Selector/5 -> PPU2CB-MCB/6  "<Inhibit>"
  PPU2CB-MCB/1 -> InputState/1
  Initialise/1 -> PPU2CB-MCB/4

== system IOControls/ForEachVehicle/IOControls/Non-CabControl/CircuitBreakersofEDB/PPU3CB ==
  note: States:
      | Tripped
      | Set
  MCBControl : Inport  OutDataTypeStr=Bus: BD_IOControls_In_MCBControl
  Initialise : Inport  Port=2
  Bus Selector : BusSelector  OutputSignals=Value,Mode,InitVal,InternalRequest,Inhibit,TripRequest
  PPU3CB-MCB : IOStateMachinesLib/MCB  InitSource=internal  InitState=InitState  OffStateValue=OffStateValue  OnStateValue=OnStateValue
      settings: SourceProductName=IO State Machines
  InputState : Outport  VectorParamsAs1DForOutWhenUnconnected=off
  MCBTripState : Outport  Port=2  VectorParamsAs1DForOutWhenUnconnected=off
  wires:
  PPU3CB-MCB/2 -> MCBTripState/1
  Bus Selector/6 -> PPU3CB-MCB/7  "<TripRequest>"
  MCBControl/1 -> Bus Selector/1
  Bus Selector/1 -> PPU3CB-MCB/1  "<Value>"
  Bus Selector/2 -> PPU3CB-MCB/2  "<Mode>"
  Bus Selector/3 -> PPU3CB-MCB/3  "<InitVal>"
  Bus Selector/4 -> PPU3CB-MCB/5  "<InternalRequest>"
  Bus Selector/5 -> PPU3CB-MCB/6  "<Inhibit>"
  PPU3CB-MCB/1 -> InputState/1
  Initialise/1 -> PPU3CB-MCB/4

== system IOControls/ForEachVehicle/IOControls/Non-CabControl/CircuitBreakersofEDB/PTCB ==
  note: States:
      | Tripped
      | Set
  MCBControl : Inport  OutDataTypeStr=Bus: BD_IOControls_In_MCBControl
  Initialise : Inport  Port=2
  Bus Selector : BusSelector  OutputSignals=Value,Mode,InitVal,InternalRequest,Inhibit,TripRequest
  PTCB-MCB : IOStateMachinesLib/MCB  InitSource=internal  InitState=InitState  OffStateValue=OffStateValue  OnStateValue=OnStateValue
      settings: SourceProductName=IO State Machines
  InputState : Outport  VectorParamsAs1DForOutWhenUnconnected=off
  MCBTripState : Outport  Port=2  VectorParamsAs1DForOutWhenUnconnected=off
  wires:
  PTCB-MCB/2 -> MCBTripState/1
  Bus Selector/6 -> PTCB-MCB/7  "<TripRequest>"
  MCBControl/1 -> Bus Selector/1
  Bus Selector/1 -> PTCB-MCB/1  "<Value>"
  Bus Selector/2 -> PTCB-MCB/2  "<Mode>"
  Bus Selector/3 -> PTCB-MCB/3  "<InitVal>"
  Bus Selector/4 -> PTCB-MCB/5  "<InternalRequest>"
  Bus Selector/5 -> PTCB-MCB/6  "<Inhibit>"
  PTCB-MCB/1 -> InputState/1
  Initialise/1 -> PTCB-MCB/4

== system IOControls/ForEachVehicle/IOControls/Non-CabControl/CircuitBreakersofEDB/RIO1CB ==
  note: States:
      | Tripped
      | Set
  MCBControl : Inport  OutDataTypeStr=Bus: BD_IOControls_In_MCBControl
  Initialise : Inport  Port=2
  Bus Selector : BusSelector  OutputSignals=Value,Mode,InitVal,InternalRequest,Inhibit,TripRequest
  RIO1CB-MCB : IOStateMachinesLib/MCB  InitSource=internal  InitState=InitState  OffStateValue=OffStateValue  OnStateValue=OnStateValue
      settings: SourceProductName=IO State Machines
  InputState : Outport  VectorParamsAs1DForOutWhenUnconnected=off
  MCBTripState : Outport  Port=2  VectorParamsAs1DForOutWhenUnconnected=off
  wires:
  RIO1CB-MCB/2 -> MCBTripState/1
  Bus Selector/6 -> RIO1CB-MCB/7  "<TripRequest>"
  MCBControl/1 -> Bus Selector/1
  Bus Selector/1 -> RIO1CB-MCB/1  "<Value>"
  Bus Selector/2 -> RIO1CB-MCB/2  "<Mode>"
  Bus Selector/3 -> RIO1CB-MCB/3  "<InitVal>"
  Bus Selector/4 -> RIO1CB-MCB/5  "<InternalRequest>"
  Bus Selector/5 -> RIO1CB-MCB/6  "<Inhibit>"
  RIO1CB-MCB/1 -> InputState/1
  Initialise/1 -> RIO1CB-MCB/4

== system IOControls/ForEachVehicle/IOControls/Non-CabControl/CircuitBreakersofEDB/RIO2CB ==
  note: States:
      | Tripped
      | Set
  MCBControl : Inport  OutDataTypeStr=Bus: BD_IOControls_In_MCBControl
  Initialise : Inport  Port=2
  Bus Selector : BusSelector  OutputSignals=Value,Mode,InitVal,InternalRequest,Inhibit,TripRequest
  RIO2CB-MCB : IOStateMachinesLib/MCB  InitSource=internal  InitState=InitState  OffStateValue=OffStateValue  OnStateValue=OnStateValue
      settings: SourceProductName=IO State Machines
  InputState : Outport  VectorParamsAs1DForOutWhenUnconnected=off
  MCBTripState : Outport  Port=2  VectorParamsAs1DForOutWhenUnconnected=off
  wires:
  RIO2CB-MCB/2 -> MCBTripState/1
  Bus Selector/6 -> RIO2CB-MCB/7  "<TripRequest>"
  MCBControl/1 -> Bus Selector/1
  Bus Selector/1 -> RIO2CB-MCB/1  "<Value>"
  Bus Selector/2 -> RIO2CB-MCB/2  "<Mode>"
  Bus Selector/3 -> RIO2CB-MCB/3  "<InitVal>"
  Bus Selector/4 -> RIO2CB-MCB/5  "<InternalRequest>"
  Bus Selector/5 -> RIO2CB-MCB/6  "<Inhibit>"
  RIO2CB-MCB/1 -> InputState/1
  Initialise/1 -> RIO2CB-MCB/4

== system IOControls/ForEachVehicle/IOControls/Non-CabControl/CircuitBreakersofEDB/RPTCB ==
  note: States:
      | Tripped
      | Set
  MCBControl : Inport  OutDataTypeStr=Bus: BD_IOControls_In_MCBControl
  Initialise : Inport  Port=2
  Bus Selector : BusSelector  OutputSignals=Value,Mode,InitVal,InternalRequest,Inhibit,TripRequest
  RPTCB-MCB : IOStateMachinesLib/MCB  InitSource=internal  InitState=InitState  OffStateValue=OffStateValue  OnStateValue=OnStateValue
      settings: SourceProductName=IO State Machines
  InputState : Outport  VectorParamsAs1DForOutWhenUnconnected=off
  MCBTripState : Outport  Port=2  VectorParamsAs1DForOutWhenUnconnected=off
  wires:
  RPTCB-MCB/2 -> MCBTripState/1
  Bus Selector/6 -> RPTCB-MCB/7  "<TripRequest>"
  MCBControl/1 -> Bus Selector/1
  Bus Selector/1 -> RPTCB-MCB/1  "<Value>"
  Bus Selector/2 -> RPTCB-MCB/2  "<Mode>"
  Bus Selector/3 -> RPTCB-MCB/3  "<InitVal>"
  Bus Selector/4 -> RPTCB-MCB/5  "<InternalRequest>"
  Bus Selector/5 -> RPTCB-MCB/6  "<Inhibit>"
  RPTCB-MCB/1 -> InputState/1
  Initialise/1 -> RPTCB-MCB/4

== system IOControls/ForEachVehicle/IOControls/Non-CabControl/CircuitBreakersofEDB/RSACB ==
  note: States:
      | Tripped
      | Set
  MCBControl : Inport  OutDataTypeStr=Bus: BD_IOControls_In_MCBControl
  Initialise : Inport  Port=2
  Bus Selector : BusSelector  OutputSignals=Value,Mode,InitVal,InternalRequest,Inhibit,TripRequest
  RSACB-MCB : IOStateMachinesLib/MCB  InitSource=internal  InitState=InitState  OffStateValue=OffStateValue  OnStateValue=OnStateValue
      settings: SourceProductName=IO State Machines
  InputState : Outport  VectorParamsAs1DForOutWhenUnconnected=off
  MCBTripState : Outport  Port=2  VectorParamsAs1DForOutWhenUnconnected=off
  wires:
  RSACB-MCB/2 -> MCBTripState/1
  Bus Selector/6 -> RSACB-MCB/7  "<TripRequest>"
  MCBControl/1 -> Bus Selector/1
  Bus Selector/1 -> RSACB-MCB/1  "<Value>"
  Bus Selector/2 -> RSACB-MCB/2  "<Mode>"
  Bus Selector/3 -> RSACB-MCB/3  "<InitVal>"
  Bus Selector/4 -> RSACB-MCB/5  "<InternalRequest>"
  Bus Selector/5 -> RSACB-MCB/6  "<Inhibit>"
  RSACB-MCB/1 -> InputState/1
  Initialise/1 -> RSACB-MCB/4

== system IOControls/ForEachVehicle/IOControls/Non-CabControl/CircuitBreakersofEDB/SAC1CCB ==
  note: States:
      | Tripped
      | Set
  MCBControl : Inport  OutDataTypeStr=Bus: BD_IOControls_In_MCBControl
  Initialise : Inport  Port=2
  Bus Selector : BusSelector  OutputSignals=Value,Mode,InitVal,InternalRequest,Inhibit,TripRequest
  SAC1CCB-MCB : IOStateMachinesLib/MCB  InitSource=internal  InitState=InitState  OffStateValue=OffStateValue  OnStateValue=OnStateValue
      settings: SourceProductName=IO State Machines
  InputState : Outport  VectorParamsAs1DForOutWhenUnconnected=off
  MCBTripState : Outport  Port=2  VectorParamsAs1DForOutWhenUnconnected=off
  wires:
  SAC1CCB-MCB/2 -> MCBTripState/1
  Bus Selector/6 -> SAC1CCB-MCB/7  "<TripRequest>"
  MCBControl/1 -> Bus Selector/1
  Bus Selector/1 -> SAC1CCB-MCB/1  "<Value>"
  Bus Selector/2 -> SAC1CCB-MCB/2  "<Mode>"
  Bus Selector/3 -> SAC1CCB-MCB/3  "<InitVal>"
  Bus Selector/4 -> SAC1CCB-MCB/5  "<InternalRequest>"
  Bus Selector/5 -> SAC1CCB-MCB/6  "<Inhibit>"
  SAC1CCB-MCB/1 -> InputState/1
  Initialise/1 -> SAC1CCB-MCB/4

== system IOControls/ForEachVehicle/IOControls/Non-CabControl/CircuitBreakersofEDB/SAC2CCB ==
  note: States:
      | Tripped
      | Set
  MCBControl : Inport  OutDataTypeStr=Bus: BD_IOControls_In_MCBControl
  Initialise : Inport  Port=2
  Bus Selector : BusSelector  OutputSignals=Value,Mode,InitVal,InternalRequest,Inhibit,TripRequest
  SAC2CCB-MCB : IOStateMachinesLib/MCB  InitSource=internal  InitState=InitState  OffStateValue=OffStateValue  OnStateValue=OnStateValue
      settings: SourceProductName=IO State Machines
  InputState : Outport  VectorParamsAs1DForOutWhenUnconnected=off
  MCBTripState : Outport  Port=2  VectorParamsAs1DForOutWhenUnconnected=off
  wires:
  SAC2CCB-MCB/2 -> MCBTripState/1
  Bus Selector/6 -> SAC2CCB-MCB/7  "<TripRequest>"
  MCBControl/1 -> Bus Selector/1
  Bus Selector/1 -> SAC2CCB-MCB/1  "<Value>"
  Bus Selector/2 -> SAC2CCB-MCB/2  "<Mode>"
  Bus Selector/3 -> SAC2CCB-MCB/3  "<InitVal>"
  Bus Selector/4 -> SAC2CCB-MCB/5  "<InternalRequest>"
  Bus Selector/5 -> SAC2CCB-MCB/6  "<Inhibit>"
  SAC2CCB-MCB/1 -> InputState/1
  Initialise/1 -> SAC2CCB-MCB/4

== system IOControls/ForEachVehicle/IOControls/Non-CabControl/CircuitBreakersofEDB/SIOCB1 ==
  note: States:
      | Tripped
      | Set
  MCBControl : Inport  OutDataTypeStr=Bus: BD_IOControls_In_MCBControl
  Initialise : Inport  Port=2
  Bus Selector : BusSelector  OutputSignals=Value,Mode,InitVal,InternalRequest,Inhibit,TripRequest
  SIOCB1-MCB : IOStateMachinesLib/MCB  InitSource=internal  InitState=InitState  OffStateValue=OffStateValue  OnStateValue=OnStateValue
      settings: SourceProductName=IO State Machines
  InputState : Outport  VectorParamsAs1DForOutWhenUnconnected=off
  MCBTripState : Outport  Port=2  VectorParamsAs1DForOutWhenUnconnected=off
  wires:
  SIOCB1-MCB/2 -> MCBTripState/1
  Bus Selector/6 -> SIOCB1-MCB/7  "<TripRequest>"
  MCBControl/1 -> Bus Selector/1
  Bus Selector/1 -> SIOCB1-MCB/1  "<Value>"
  Bus Selector/2 -> SIOCB1-MCB/2  "<Mode>"
  Bus Selector/3 -> SIOCB1-MCB/3  "<InitVal>"
  Bus Selector/4 -> SIOCB1-MCB/5  "<InternalRequest>"
  Bus Selector/5 -> SIOCB1-MCB/6  "<Inhibit>"
  SIOCB1-MCB/1 -> InputState/1
  Initialise/1 -> SIOCB1-MCB/4

== system IOControls/ForEachVehicle/IOControls/Non-CabControl/CircuitBreakersofEDB/SIOCB2 ==
  note: States:
      | Tripped
      | Set
  MCBControl : Inport  OutDataTypeStr=Bus: BD_IOControls_In_MCBControl
  Initialise : Inport  Port=2
  Bus Selector : BusSelector  OutputSignals=Value,Mode,InitVal,InternalRequest,Inhibit,TripRequest
  SIOCB2-MCB : IOStateMachinesLib/MCB  InitSource=internal  InitState=InitState  OffStateValue=OffStateValue  OnStateValue=OnStateValue
      settings: SourceProductName=IO State Machines
  InputState : Outport  VectorParamsAs1DForOutWhenUnconnected=off
  MCBTripState : Outport  Port=2  VectorParamsAs1DForOutWhenUnconnected=off
  wires:
  SIOCB2-MCB/2 -> MCBTripState/1
  Bus Selector/6 -> SIOCB2-MCB/7  "<TripRequest>"
  MCBControl/1 -> Bus Selector/1
  Bus Selector/1 -> SIOCB2-MCB/1  "<Value>"
  Bus Selector/2 -> SIOCB2-MCB/2  "<Mode>"
  Bus Selector/3 -> SIOCB2-MCB/3  "<InitVal>"
  Bus Selector/4 -> SIOCB2-MCB/5  "<InternalRequest>"
  Bus Selector/5 -> SIOCB2-MCB/6  "<Inhibit>"
  SIOCB2-MCB/1 -> InputState/1
  Initialise/1 -> SIOCB2-MCB/4

== system IOControls/ForEachVehicle/IOControls/Non-CabControl/CircuitBreakersofEDB/SOCB1 ==
  note: States:
      | Tripped
      | Set
  MCBControl : Inport  OutDataTypeStr=Bus: BD_IOControls_In_MCBControl
  Initialise : Inport  Port=2
  Bus Selector : BusSelector  OutputSignals=Value,Mode,InitVal,InternalRequest,Inhibit,TripRequest
  SOCB1-MCB : IOStateMachinesLib/MCB  InitSource=internal  InitState=InitState  OffStateValue=OffStateValue  OnStateValue=OnStateValue
      settings: SourceProductName=IO State Machines
  InputState : Outport  VectorParamsAs1DForOutWhenUnconnected=off
  MCBTripState : Outport  Port=2  VectorParamsAs1DForOutWhenUnconnected=off
  wires:
  SOCB1-MCB/2 -> MCBTripState/1
  Bus Selector/6 -> SOCB1-MCB/7  "<TripRequest>"
  MCBControl/1 -> Bus Selector/1
  Bus Selector/1 -> SOCB1-MCB/1  "<Value>"
  Bus Selector/2 -> SOCB1-MCB/2  "<Mode>"
  Bus Selector/3 -> SOCB1-MCB/3  "<InitVal>"
  Bus Selector/4 -> SOCB1-MCB/5  "<InternalRequest>"
  Bus Selector/5 -> SOCB1-MCB/6  "<Inhibit>"
  SOCB1-MCB/1 -> InputState/1
  Initialise/1 -> SOCB1-MCB/4

== system IOControls/ForEachVehicle/IOControls/Non-CabControl/CircuitBreakersofEDB/SOCB2 ==
  note: States:
      | Tripped
      | Set
  MCBControl : Inport  OutDataTypeStr=Bus: BD_IOControls_In_MCBControl
  Initialise : Inport  Port=2
  Bus Selector : BusSelector  OutputSignals=Value,Mode,InitVal,InternalRequest,Inhibit,TripRequest
  SOCB2-MCB : IOStateMachinesLib/MCB  InitSource=internal  InitState=InitState  OffStateValue=OffStateValue  OnStateValue=OnStateValue
      settings: SourceProductName=IO State Machines
  InputState : Outport  VectorParamsAs1DForOutWhenUnconnected=off
  MCBTripState : Outport  Port=2  VectorParamsAs1DForOutWhenUnconnected=off
  wires:
  SOCB2-MCB/2 -> MCBTripState/1
  Bus Selector/6 -> SOCB2-MCB/7  "<TripRequest>"
  MCBControl/1 -> Bus Selector/1
  Bus Selector/1 -> SOCB2-MCB/1  "<Value>"
  Bus Selector/2 -> SOCB2-MCB/2  "<Mode>"
  Bus Selector/3 -> SOCB2-MCB/3  "<InitVal>"
  Bus Selector/4 -> SOCB2-MCB/5  "<InternalRequest>"
  Bus Selector/5 -> SOCB2-MCB/6  "<Inhibit>"
  SOCB2-MCB/1 -> InputState/1
  Initialise/1 -> SOCB2-MCB/4

== system IOControls/ForEachVehicle/IOControls/Non-CabControl/CircuitBreakersofEDB/SP11CB ==
  note: States:
      | Tripped
      | Set
  MCBControl : Inport  OutDataTypeStr=Bus: BD_IOControls_In_MCBControl
  Initialise : Inport  Port=2
  Bus Selector : BusSelector  OutputSignals=Value,Mode,InitVal,InternalRequest,Inhibit,TripRequest
  SP11CB-MCB : IOStateMachinesLib/MCB  InitSource=internal  InitState=InitState  OffStateValue=OffStateValue  OnStateValue=OnStateValue
      settings: SourceProductName=IO State Machines
  InputState : Outport  VectorParamsAs1DForOutWhenUnconnected=off
  MCBTripState : Outport  Port=2  VectorParamsAs1DForOutWhenUnconnected=off
  wires:
  SP11CB-MCB/2 -> MCBTripState/1
  Bus Selector/6 -> SP11CB-MCB/7  "<TripRequest>"
  MCBControl/1 -> Bus Selector/1
  Bus Selector/1 -> SP11CB-MCB/1  "<Value>"
  Bus Selector/2 -> SP11CB-MCB/2  "<Mode>"
  Bus Selector/3 -> SP11CB-MCB/3  "<InitVal>"
  Bus Selector/4 -> SP11CB-MCB/5  "<InternalRequest>"
  Bus Selector/5 -> SP11CB-MCB/6  "<Inhibit>"
  SP11CB-MCB/1 -> InputState/1
  Initialise/1 -> SP11CB-MCB/4

== system IOControls/ForEachVehicle/IOControls/Non-CabControl/CircuitBreakersofEDB/SP12CB ==
  note: States:
      | Tripped
      | Set
  MCBControl : Inport  OutDataTypeStr=Bus: BD_IOControls_In_MCBControl
  Initialise : Inport  Port=2
  Bus Selector : BusSelector  OutputSignals=Value,Mode,InitVal,InternalRequest,Inhibit,TripRequest
  SP12CB-MCB : IOStateMachinesLib/MCB  InitSource=internal  InitState=InitState  OffStateValue=OffStateValue  OnStateValue=OnStateValue
      settings: SourceProductName=IO State Machines
  InputState : Outport  VectorParamsAs1DForOutWhenUnconnected=off
  MCBTripState : Outport  Port=2  VectorParamsAs1DForOutWhenUnconnected=off
  wires:
  SP12CB-MCB/2 -> MCBTripState/1
  Bus Selector/6 -> SP12CB-MCB/7  "<TripRequest>"
  MCBControl/1 -> Bus Selector/1
  Bus Selector/1 -> SP12CB-MCB/1  "<Value>"
  Bus Selector/2 -> SP12CB-MCB/2  "<Mode>"
  Bus Selector/3 -> SP12CB-MCB/3  "<InitVal>"
  Bus Selector/4 -> SP12CB-MCB/5  "<InternalRequest>"
  Bus Selector/5 -> SP12CB-MCB/6  "<Inhibit>"
  SP12CB-MCB/1 -> InputState/1
  Initialise/1 -> SP12CB-MCB/4

== system IOControls/ForEachVehicle/IOControls/Non-CabControl/CircuitBreakersofEDB/SP1CB ==
  note: States:
      | Tripped
      | Set
  MCBControl : Inport  OutDataTypeStr=Bus: BD_IOControls_In_MCBControl
  Initialise : Inport  Port=2
  Bus Selector : BusSelector  OutputSignals=Value,Mode,InitVal,InternalRequest,Inhibit,TripRequest
  SP1CB-MCB : IOStateMachinesLib/MCB  InitSource=internal  InitState=InitState  OffStateValue=OffStateValue  OnStateValue=OnStateValue
      settings: SourceProductName=IO State Machines
  InputState : Outport  VectorParamsAs1DForOutWhenUnconnected=off
  MCBTripState : Outport  Port=2  VectorParamsAs1DForOutWhenUnconnected=off
  wires:
  SP1CB-MCB/2 -> MCBTripState/1
  Bus Selector/6 -> SP1CB-MCB/7  "<TripRequest>"
  MCBControl/1 -> Bus Selector/1
  Bus Selector/1 -> SP1CB-MCB/1  "<Value>"
  Bus Selector/2 -> SP1CB-MCB/2  "<Mode>"
  Bus Selector/3 -> SP1CB-MCB/3  "<InitVal>"
  Bus Selector/4 -> SP1CB-MCB/5  "<InternalRequest>"
  Bus Selector/5 -> SP1CB-MCB/6  "<Inhibit>"
  SP1CB-MCB/1 -> InputState/1
  Initialise/1 -> SP1CB-MCB/4

== system IOControls/ForEachVehicle/IOControls/Non-CabControl/CircuitBreakersofEDB/SP2CB ==
  note: States:
      | Tripped
      | Set
  MCBControl : Inport  OutDataTypeStr=Bus: BD_IOControls_In_MCBControl
  Initialise : Inport  Port=2
  Bus Selector : BusSelector  OutputSignals=Value,Mode,InitVal,InternalRequest,Inhibit,TripRequest
  SP2CB-MCB : IOStateMachinesLib/MCB  InitSource=internal  InitState=InitState  OffStateValue=OffStateValue  OnStateValue=OnStateValue
      settings: SourceProductName=IO State Machines
  InputState : Outport  VectorParamsAs1DForOutWhenUnconnected=off
  MCBTripState : Outport  Port=2  VectorParamsAs1DForOutWhenUnconnected=off
  wires:
  SP2CB-MCB/2 -> MCBTripState/1
  Bus Selector/6 -> SP2CB-MCB/7  "<TripRequest>"
  MCBControl/1 -> Bus Selector/1
  Bus Selector/1 -> SP2CB-MCB/1  "<Value>"
  Bus Selector/2 -> SP2CB-MCB/2  "<Mode>"
  Bus Selector/3 -> SP2CB-MCB/3  "<InitVal>"
  Bus Selector/4 -> SP2CB-MCB/5  "<InternalRequest>"
  Bus Selector/5 -> SP2CB-MCB/6  "<Inhibit>"
  SP2CB-MCB/1 -> InputState/1
  Initialise/1 -> SP2CB-MCB/4

== system IOControls/ForEachVehicle/IOControls/Non-CabControl/CircuitBreakersofEDB/SP3CB ==
  note: States:
      | Tripped
      | Set
  MCBControl : Inport  OutDataTypeStr=Bus: BD_IOControls_In_MCBControl
  Initialise : Inport  Port=2
  Bus Selector : BusSelector  OutputSignals=Value,Mode,InitVal,InternalRequest,Inhibit,TripRequest
  SP3CB-MCB : IOStateMachinesLib/MCB  InitSource=internal  InitState=InitState  OffStateValue=OffStateValue  OnStateValue=OnStateValue
      settings: SourceProductName=IO State Machines
  InputState : Outport  VectorParamsAs1DForOutWhenUnconnected=off
  MCBTripState : Outport  Port=2  VectorParamsAs1DForOutWhenUnconnected=off
  wires:
  SP3CB-MCB/2 -> MCBTripState/1
  Bus Selector/6 -> SP3CB-MCB/7  "<TripRequest>"
  MCBControl/1 -> Bus Selector/1
  Bus Selector/1 -> SP3CB-MCB/1  "<Value>"
  Bus Selector/2 -> SP3CB-MCB/2  "<Mode>"
  Bus Selector/3 -> SP3CB-MCB/3  "<InitVal>"
  Bus Selector/4 -> SP3CB-MCB/5  "<InternalRequest>"
  Bus Selector/5 -> SP3CB-MCB/6  "<Inhibit>"
  SP3CB-MCB/1 -> InputState/1
  Initialise/1 -> SP3CB-MCB/4
